simulink model "Lidar_System_July7"  (Simulink 7.3)
settings: Solver=FixedStepDiscrete  StartTime=0.0  StopTime=inf  FixedStep=0.1  MaxStep=0.2  RelTol=1e-3
libraries: dspmtrx3 x3, simulink x2, vipstatistics x2, dspstat3 x2, vipgeotforms x1
(part 1 of 3)
settings Model: Creator=gclayton  LastModifiedBy=wildcat
settings DebuggingCC: InheritedTsInSrcMsg=none
settings RTWCC: SystemTargetFile=rlnx.tlc  GenCodeOnly=on  TemplateMakefile=rlnx_ubuntu.tmf  Description=Linux Real-Time Target  ProcessScript=rlnx_make_rtw_hook
settings RTWCC: CustomInclude=|
  | /usr/local/include/opencv/
  | /usr/local/include/
settings CodeAppCC: GenerateComments=off  SimulinkBlockComments=off
settings STFCustomTargetCC: ModelReferenceCompliant=off  MatFileLogging=on  SystemTargetFile=rlnx.tlc
settings GRTTargetCC: ModelReferenceCompliant=off  ParMdlRefBuildCompliant=off  CompOptLevelCompliant=off
settings CustomProperty: DataType=string  Value="-lm -ldl /usr/local/lib/libopencv_highgui.so.2.4 /usr/local/lib/libopencv_core.so.2.4 /usr/local/lib/libopencv_imgproc.so.2.4  -lc_urg -lc_urg_connection -lc_urg_system -lphidget21"
settings EnumStrPairs: String=PC

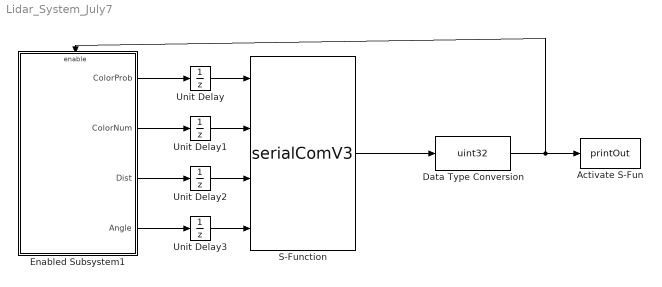
== system Lidar_System_July7 ==
  Activate S-Fun : S-Function  FunctionName=printOut  EnableBusSupport=off
  Data Type Conversion : DataTypeConversion  OutDataTypeMode=uint32  OutDataType=fixdt(1, 16)  OutScaling=2^0  OutDataTypeStr=uint32
  Enabled Subsystem1 : Subsystem  TreatAsAtomicUnit=on
  S-Function : S-Function  FunctionName=serialComV3  EnableBusSupport=off
  Unit Delay : UnitDelay  SampleTime=-1
  Unit Delay1 : UnitDelay  X0=int32(0)  SampleTime=-1
  Unit Delay2 : UnitDelay  X0=int32(0)  SampleTime=-1
  Unit Delay3 : UnitDelay  X0=int32(0)  SampleTime=-1
  wires:
  S-Function/1 -> Data Type Conversion/1
  Enabled Subsystem1/1(ColorProb) -> Unit Delay/1
  Enabled Subsystem1/2(ColorNum) -> Unit Delay1/1
  Enabled Subsystem1/3(Dist) -> Unit Delay2/1
  Enabled Subsystem1/4(Angle) -> Unit Delay3/1
  Unit Delay/1 -> S-Function/1
  Unit Delay1/1 -> S-Function/2
  Unit Delay2/1 -> S-Function/3
  Unit Delay3/1 -> S-Function/4
  Data Type Conversion/1 -> Activate S-Fun/1, Enabled Subsystem1/Enable

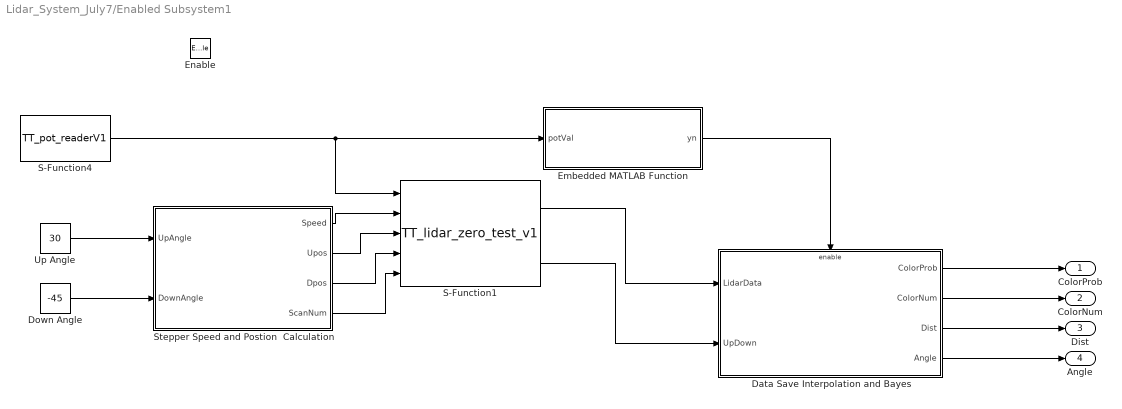
== system Lidar_System_July7/Enabled Subsystem1 ==
  Enable : EnablePort
  Data Save Interpolation and Bayes : Subsystem  TreatAsAtomicUnit=on
  Down Angle : Constant  Value=-45  OutDataType=fixdt(1, 16)  OutScaling=2^0
  Embedded MATLAB Function : Stateflow chart
  S-Function1 : S-Function  FunctionName=TT_lidar_zero_test_v1  EnableBusSupport=off
  S-Function4 : S-Function  FunctionName=TT_pot_readerV1  EnableBusSupport=off
  Stepper Speed and Postion  Calculation : Stateflow chart
  Up Angle : Constant  Value=30  OutDataType=fixdt(1, 16)  OutScaling=2^0
  ColorProb : Outport  OutDataType=fixdt(1, 16)  OutScaling=2^0
  ColorNum : Outport  Port=2  OutDataType=fixdt(1, 16)  OutScaling=2^0
  Dist : Outport  Port=3  OutDataType=fixdt(1, 16)  OutScaling=2^0
  Angle : Outport  Port=4  OutDataType=fixdt(1, 16)  OutScaling=2^0
  wires:
  S-Function4/1 -> S-Function1/1, Embedded MATLAB Function/1(potVal)
  Stepper Speed and Postion  Calculation/1(Speed) -> S-Function1/2
  Stepper Speed and Postion  Calculation/2(Upos) -> S-Function1/3
  Stepper Speed and Postion  Calculation/3(Dpos) -> S-Function1/4
  Stepper Speed and Postion  Calculation/4(ScanNum) -> S-Function1/5
  Embedded MATLAB Function/1(yn) -> Data Save Interpolation and Bayes/Enable
  S-Function1/1 -> Data Save Interpolation and Bayes/1(LidarData)
  S-Function1/2 -> Data Save Interpolation and Bayes/2(UpDown)
  Data Save Interpolation and Bayes/1(ColorProb) -> ColorProb/1
  Data Save Interpolation and Bayes/2(ColorNum) -> ColorNum/1
  Data Save Interpolation and Bayes/3(Dist) -> Dist/1
  Data Save Interpolation and Bayes/4(Angle) -> Angle/1
  Down Angle/1 -> Stepper Speed and Postion  Calculation/2(DownAngle)
  Up Angle/1 -> Stepper Speed and Postion  Calculation/1(UpAngle)

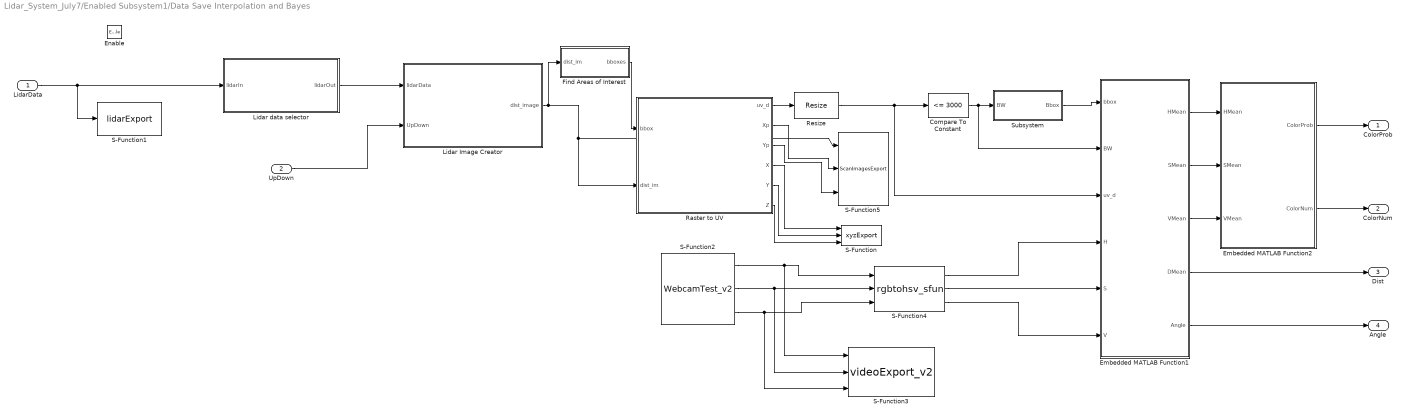
== system Lidar_System_July7/Enabled Subsystem1/Data Save Interpolation and Bayes ==
  LidarData : Inport  OutDataType=fixdt(1, 16)  OutScaling=2^0
  UpDown : Inport  Port=2  OutDataType=fixdt(1, 16)  OutScaling=2^0
  Enable : EnablePort
  Compare To Constant : simulink/Logic and Bit Operations/Compare To Constant  SystemSampleTime=-1  relop=<=  const=3000  LogicOutDataTypeMode=boolean  ZeroCross=off
  Embedded MATLAB Function1 : Stateflow chart
  Embedded MATLAB Function2 : Stateflow chart
  Find Areas of Interest : Subsystem
  Lidar Image Creator : Stateflow chart
  Lidar data selector : Stateflow chart
  Raster to UV : Stateflow chart
  Resize : vipgeotforms/Resize  DialogController=vipDDGCreate  DialogControllerArgs=DataTag2  specify=Number of output rows and columns  rfactor=[200 150]  outCols=25  outRows=25  outRowsCols=[480 640]  interp_method=Bilinear  antialias=on  useROI=off  roiFlag=off  prodOutputMode=Binary point scaling  prodOutputWordLength=32  prodOutputFracLength=10  roundingMode=Nearest  overflowMode=on
  S-Function : S-Function  FunctionName=xyzExport  EnableBusSupport=off
  S-Function1 : S-Function  FunctionName=lidarExport  EnableBusSupport=off
  S-Function2 : S-Function  FunctionName=WebcamTest_v2  EnableBusSupport=off
  S-Function3 : S-Function  FunctionName=videoExport_v2  EnableBusSupport=off
  S-Function4 : S-Function  FunctionName=rgbtohsv_sfun  EnableBusSupport=off
  S-Function5 : S-Function  FunctionName=ScanImagesExport  EnableBusSupport=off
  Subsystem : Subsystem
  ColorProb : Outport  OutDataType=fixdt(1, 16)  OutScaling=2^0
  ColorNum : Outport  Port=2  OutDataType=fixdt(1, 16)  OutScaling=2^0
  Dist : Outport  Port=3  OutDataType=fixdt(1, 16)  OutScaling=2^0
  Angle : Outport  Port=4  OutDataType=fixdt(1, 16)  OutScaling=2^0
  wires:
  Lidar data selector/1(lidarOut) -> Lidar Image Creator/1(lidarData)
  UpDown/1 -> Lidar Image Creator/2(UpDown)
  Lidar Image Creator/1(dist_image) -> Find Areas of Interest/1(dist_im), Raster to UV/2(dist_im), S-Function5/1
  Find Areas of Interest/1(bboxes) -> Raster to UV/1(bbox)
  Compare To Constant/1 -> Subsystem/1(BW), Embedded MATLAB Function1/2(BW)
  Subsystem/1(Bbox) -> Embedded MATLAB Function1/1(bbox)
  Embedded MATLAB Function1/3(VMean) -> Embedded MATLAB Function2/3(VMean)
  Embedded MATLAB Function1/2(SMean) -> Embedded MATLAB Function2/2(SMean)
  Embedded MATLAB Function1/1(HMean) -> Embedded MATLAB Function2/1(HMean)
  Raster to UV/1(uv_d) -> Resize/1
  Embedded MATLAB Function2/1(ColorProb) -> ColorProb/1
  Embedded MATLAB Function2/2(ColorNum) -> ColorNum/1
  Embedded MATLAB Function1/5(Angle) -> Angle/1
  Embedded MATLAB Function1/4(DMean) -> Dist/1
  S-Function2/1 -> S-Function4/1, S-Function3/1
  S-Function2/2 -> S-Function4/2, S-Function3/2
  S-Function2/3 -> S-Function4/3, S-Function3/3
  S-Function4/1 -> Embedded MATLAB Function1/4(H)
  S-Function4/2 -> Embedded MATLAB Function1/5(S)
  S-Function4/3 -> Embedded MATLAB Function1/6(V)
  LidarData/1 -> Lidar data selector/1(lidarIn), S-Function1/1
  Resize/1 -> Compare To Constant/1, Embedded MATLAB Function1/3(uv_d)
  Raster to UV/2(Xp) -> S-Function5/2
  Raster to UV/4(X) -> S-Function/1
  Raster to UV/5(Y) -> S-Function/2
  Raster to UV/6(Z) -> S-Function/3
  Raster to UV/3(Yp) -> S-Function5/3

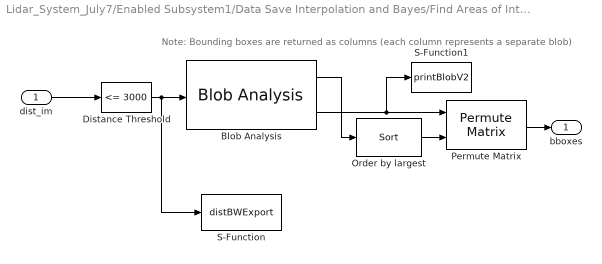
== system Lidar_System_July7/Enabled Subsystem1/Data Save Interpolation and Bayes/Find Areas of Interest ==
  note: Note: Bounding boxes are returned as columns (each column represents a separate blob)
  dist_im : Inport  OutDataType=fixdt(1, 16)  OutScaling=2^0
  Blob Analysis : vipstatistics/Blob Analysis  DialogController=vipDDGCreate  DialogControllerArgs=DataTag0  area=on  centroid=off  bBox=on  majorAxis=off  minorAxis=off  angle=off  eccentricity=off  equivDiameterSq=off  extent=off  perimeter=off  maxBlobs=8  warnIfNumBlobsExceeded=on  isCount=off  useMinArea=on  minArea=30  useMaxArea=off  maxArea=intmax('uint32')  excludeBorderBlob=off  outDT=double  isOutVarDim=off  isFill=on  fillValues=-1  conn=8  isLabel=off  outputMode=Binary point scaling  outputWordLength=32  outputFracLength=16  firstCoeffMode=Binary point scaling  firstCoeffWordLength=16  firstCoeffFracLength=14  secondCoeffMode=Binary point scaling  secondCoeffWordLength=32  secondCoeffFracLength=16  accumMode=Binary point scaling  accumWordLength=32  accumFracLength=0  prodOutputMode=Binary point scaling  prodOutputWordLength=32  prodOutputFracLength=16  roundingMode=Floor  overflowMode=off
  Distance Threshold : simulink/Logic and Bit Operations/Compare To Constant  SystemSampleTime=-1  relop=<=  const=3000  LogicOutDataTypeMode=boolean  ZeroCross=off
  Order by largest : dspstat3/Sort  DialogController=dspDDGCreate  DialogControllerArgs=DataTag1  otype=Index  dir=Descending  sortAlg=Quick sort  roundingMode=Floor  overflowMode=off
  Permute Matrix : dspmtrx3/Permute Matrix  mode=Columns  ZeroOneIdxMode=One-based  errmode=Clip index  checkDims=off
  S-Function : S-Function  FunctionName=distBWExport  EnableBusSupport=off
  S-Function1 : S-Function  FunctionName=printBlobV2  EnableBusSupport=off
  bboxes : Outport  OutDataType=fixdt(1, 16)  OutScaling=2^0
  wires:
  dist_im/1 -> Distance Threshold/1
  Distance Threshold/1 -> Blob Analysis/1, S-Function/1
  Blob Analysis/2 -> Permute Matrix/1, S-Function1/1
  Order by largest/1 -> Permute Matrix/2
  Blob Analysis/1 -> Order by largest/1
  Permute Matrix/1 -> bboxes/1

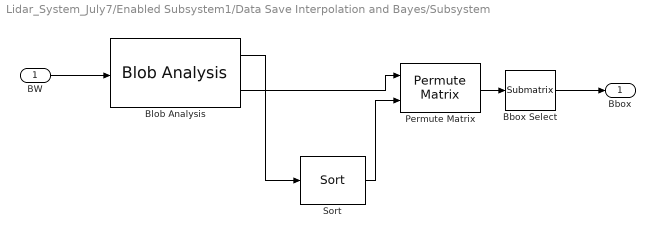
== system Lidar_System_July7/Enabled Subsystem1/Data Save Interpolation and Bayes/Subsystem ==
  BW : Inport  OutDataType=fixdt(1, 16)  OutScaling=2^0
  Bbox Select : dspmtrx3/Submatrix  RowSpan=All rows  RowStartMode=First  RowStartIndex=1  RowEndMode=Last  RowEndIndex=1  ColSpan=One column  ColStartMode=First  ColStartIndex=1  ColEndMode=Last  ColEndIndex=1
  Blob Analysis : vipstatistics/Blob Analysis  DialogController=vipDDGCreate  DialogControllerArgs=DataTag3  area=on  centroid=off  bBox=on  majorAxis=off  minorAxis=off  angle=off  eccentricity=off  equivDiameterSq=off  extent=off  perimeter=off  maxBlobs=20  warnIfNumBlobsExceeded=on  isCount=off  useMinArea=on  minArea=20  useMaxArea=off  maxArea=intmax('uint32')  excludeBorderBlob=off  outDT=double  isOutVarDim=off  isFill=on  fillValues=-1  conn=8  isLabel=off  outputMode=Binary point scaling  outputWordLength=32  outputFracLength=16  firstCoeffMode=Binary point scaling  firstCoeffWordLength=16  firstCoeffFracLength=14  secondCoeffMode=Binary point scaling  secondCoeffWordLength=32  secondCoeffFracLength=16  accumMode=Binary point scaling  accumWordLength=32  accumFracLength=0  prodOutputMode=Binary point scaling  prodOutputWordLength=32  prodOutputFracLength=16  roundingMode=Floor  overflowMode=off
  Permute Matrix : dspmtrx3/Permute Matrix  mode=Columns  ZeroOneIdxMode=One-based  errmode=Clip index  checkDims=off
  Sort : dspstat3/Sort  DialogController=dspDDGCreate  DialogControllerArgs=DataTag4  otype=Index  dir=Descending  sortAlg=Quick sort  roundingMode=Floor  overflowMode=off
  Bbox : Outport  OutDataType=fixdt(1, 16)  OutScaling=2^0
  wires:
  BW/1 -> Blob Analysis/1
  Blob Analysis/1 -> Sort/1
  Sort/1 -> Permute Matrix/2
  Blob Analysis/2 -> Permute Matrix/1
  Permute Matrix/1 -> Bbox Select/1
  Bbox Select/1 -> Bbox/1

== matlab function Enabled Subsystem1/Data Save Interpolation and Bayes/Embedded MATLAB Function1 ==
  data: bbox input double; HMean output double; BW input double; uv_d input double; H input double; S input double; V input double; SMean output double; VMean output double; DMean output double; Angle output double
function [HMean, SMean, VMean, DMean, Angle] = bbox_hist(bbox, BW, uv_d, H, S, V)
%This function creates a histogram of the color region of a detected object
%identified in a binary image within a bounding box

%Initialize variables
pixels = 0;
DRunAve = 0;
HRunAve = 0;
SRunAve = 0;
VRunAve = 0;
CDist = 0;
FoV = 62;

%Parse bbox data
left = bbox(2) + 1;
right = left + bbox(4) - 1;
bottom = bbox(1) + 1;
top = bottom + bbox(3) - 1;
Angle = int32((left + bbox(4)/2-320)/320*FoV/2);

%Check to see if valid bbox is found
if left~=-1
    %Scan the detected region of the binary image and generate histograms
    for j=left:right
        for i=bottom:top
            if BW(i,j) == 1
                pixels = pixels + 1;
                DRunAve = ((pixels-1)/pixels)*DRunAve + (1/pixels)*double(uv_d(i,j));
                HRunAve = ((pixels-1)/pixels)*HRunAve + (1/pixels)*double(H(i,j));
                SRunAve = ((pixels-1)/pixels)*SRunAve + (1/pixels)*double(S(i,j));
                VRunAve = ((pixels-1)/pixels)*VRunAve + (1/pixels)*double(V(i,j));
            end
        end
    end
    %CDist = uv_d(left,right);
end

%Means must be integers to use in Bayes Filter
DMean = int32(DRunAve/10);
%DMean = int32(CDist);
HMean = uint8(HRunAve);
SMean = uint8(SRunAve);
VMean = uint8(VRunAve);

end
